simulink model "BMW"  (R2019b)
settings: Solver=VariableStepAuto  StartTime=0.0  StopTime=20  EnableMultiTasking=on
InitFcn:
  | % Modelisation de la Machine Synchrone
  | 
  | % Constantes
  | 
  | Rs = 0.001;
  | Rdd = 0.01 ;
  | Rdq = Rdd ;
  | Rf = 7 ;
  | Ld = 1.59e-2 ;
  | Lq = Ld ;
  | Lf = 7 ;
  | Ldd = 7e-4 ;
  | Ldq = Ldd ;
  | Maf = 0.259 ;
  | Madd = 2.5e-3 ;
  | Madq = Madd ;
  | Mfdd = 6.8e-2 ;
  | npp = 2 ;
  | J = 0.1 ;
  | 
  | m = 1.8e3;
  | g = 9.81;
  | Cr = 0.3;
  | rho = 1.225;
  | S = 2.25;
  | tau = 9.65;
  | Cx = 0.3;
  | Rw = 24.13e-2;
  | 
  | Jeq = 1;
  | feq = 1;
  | 
  | K = 0.5;
  | phi = 0.5;
  | 
  | w = 2*pi*50 ;
  | 
  | Omega = w/npp ;
  | 
  | 
  | % Matrices
  | 
  | % V = [Vd Vq 0 0 Vf] ;
  | 
  | % I = [Id Iq Idd Idq If] ;
  | 
  | % F = [Fd Fq Fdd Fdq Ff] ;
  | 
  | L = [ Ld			0		Madd		0			Maf ;
  |       0			Lq		0			Madq		0 			;
  |       1.5*Madd	0		Ldd		0			Mfdd ;
  |       0        1.5*Madq			0			Ldq	0 ;
  |       1.5*Maf	0		Mfdd		0			Lf ] ;
  | 
  | L1 = inv(L) ;
  | 
  | R = [ Rs 0  0   0   0 ;
  |       0  Rs 0   0   0 ;
  |       0  0  Rdd 0   0 ;
  |       0  0  0   Rdq 0 ;
  |       0  0  0   0   Rf ] ;
  | 
  | D = [ 0 -1 0 0 0 ;
  |        1  0 0 0 0 ;
  |        0  0 0 0 0 ;
  |        0  0 0 0 0 ;
  |        0  0 0 0 0 ] ;
  | 
  |     Cl = (1/3)*[ 2  -1      -1 ;
  |      	  	        0  sqrt(3) -sqrt(3) ;
  |                   1  1       1 ] ;
  | 
  |      Cl1 = inv(Cl);
  | 
  | 
  | 
  | Clark=2/3*[	1		-1/2		-1/2
  | 	        0		sqrt(3)/2	-sqrt(3)/2
  | 	        1/2		1/2		1/2		]
  | 
  | InvClark=inv(Clark)
  | 
  | LVIDE=[Ldd   Mfdd
  |         Mfdd    Lf];
  | L2=inv(LVIDE);
  | RVIDE=[Rdd   0
  |         0    Rf];
undefined symbols (not defined in the file or in its folder): sigbuilder_block
libraries: fl_lib x12, nesl_utility x9, sdl_lib x6, simulink x4
settings Model: Creator=arzande  LastModifiedBy=jpcanesin
settings SolverCC: ZeroCrossAlgorithm=Adaptive
settings DataIOCC: LimitDataPoints=on  SaveFormat=Array  SignalLoggingSaveFormat=ModelDataLogs  ReturnWorkspaceOutputs=off
settings OptimizationCC: ExpressionDepthLimit=2147483647  InitFltsAndDblsToZero=on  LifeSpan=inf
settings DebuggingCC: UnderspecifiedInitializationDetection=Classic  MergeDetectMultiDrivingBlocksExec=none  IgnoredZcDiagnostic=none  SolverPrmCheckMsg=warning  FcnCallInpInsideContextMsg=warning  AllowSymbolicDim=off  StateNameClashWarn=warning  SFUnexpectedBacktrackingDiag=warning  SFNoUnconditionalDefaultTransitionDiag=warning  SFExecutionAtInitializationDiag=none  ArithmeticOperatorsInVariantConditions=warning
settings HardwareCC: ProdBitPerPointer=32  ProdBitPerSizeT=32  ProdBitPerPtrDiffT=32  ProdLargestAtomicFloat=None  ProdIntDivRoundTo=Undefined  ProdEndianess=Unspecified  ProdWordSize=32  ProdHWDeviceType=32-bit Generic
settings ModelReferenceCC: PropagateSignalLabelsOutOfModel=off
settings SFSimCC: SimUseLocalCustomCode=off  CustomCodeUndefinedFunction=UseInterfaceOnly
settings RTWCC: RTWUseLocalCustomCode=off
settings CodeAppCC: StateflowObjectComments=on
settings GRTTargetCC: TargetLangStandard=C89/C90 (ANSI)  GeneratePreprocessorConditionals=Disable all  CombineOutputUpdateFcns=off  GRTInterface=on
settings ConfigComp: CovMetricSettings=dw  CovHtmlReporting=on  CovSaveCumulativeToWorkspaceVar=on  CovSaveSingleToWorkspaceVar=on  CovExternalEMLEnable=off

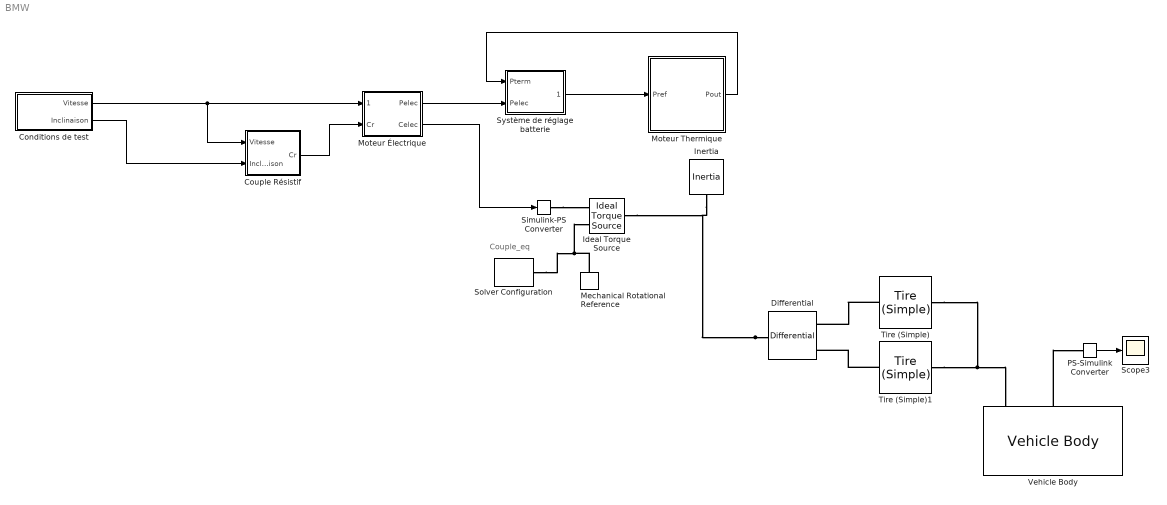
== system BMW ==
  note: Couple_eq
  Conditions de test : Subsystem  Tag=STV Subsys  LoadFcn=sigbuilder_block('load');  StartFcn=sigbuilder_block('start');  StopFcn=sigbuilder_block('stop');  ClipboardFcn=sigbuilder_block('clipboard');  mask(Sigbuilder block){tuvar=[0:10]}
      mask help: Simulink:masks:SigbuilderBlock_MD
      mask init:
      | if ~strcmp(get_param(bdroot(gcbh),'SimulationStatus'),'stopped') tuvar = sigbuilder_block('maskInit'); end
      settings: CopyFcn=sigbuilder_block('copy');  DeleteFcn=sigbuilder_block('delete');  ModelCloseFcn=sigbuilder_block('modelClose');  PreSaveFcn=sigbuilder_block('preSave');  PauseFcn=sigbuilder_block('pause');  ContinueFcn=sigbuilder_block('continue');  NameChangeFcn=sigbuilder_block('namechange');  OpenFcn=sigbuilder_block('open',[0 0 1396 804 ]);  CloseFcn=sigbuilder_block('close');
      mask Display: plot(0, 0, 100, 100,[2, 2, 32, 32, 2], [68, 8, 8, 68, 68],[32, 2], [38, 38], [32, 19, 2],[53, 60, 44], [32, 17, 17, 2],[16, 16, 31, 31]);txt = getActiveGroup(gcbh);text(2, 100, txt,'verticalAlignment', 'top');
  Couple Résistif : Subsystem
  Differential : sdl_lib/Gears/Differential  driveshaft_location=2  cd_ratio=4  friction_model=1  efficiency=[.85, .92]  mu_visc=[0, 0] N*m/(rad/s)  pwr_thr=[.001, .001] W  carrier_inertia=0 kg*m^2  planet_inertia=0 kg*m^2  temperature_TLU=[280, 300, 320] K  efficiency_ss_TLU=[.95, .9, .85]  efficiency_cd_TLU=[.95, .9, .85]  thermal_mass=50 J/K  T_init=300 K
      settings: SourceProductName=Simscape Driveline  SourceProductBaseCode=LD
  Ideal Torque Source : fl_lib/Mechanical/Mechanical Sources/Ideal Torque Source
  Inertia : fl_lib/Mechanical/Rotational Elements/Inertia  inertia=0.01 kg*m^2  w_specify=off  w_priority=High  w=0 rad/s  w_nominal_specify=off  w_nominal_unit=rad/s  w_nominal_value=1  t_specify=off  t_priority=None  t=0 N*m  t_nominal_specify=off  t_nominal_unit=N*m  t_nominal_value=1
  Mechanical Rotational Reference : fl_lib/Mechanical/Rotational Elements/Mechanical Rotational Reference
  Moteur Thermique : Subsystem
  Moteur Électrique : Subsystem
  PS-Simulink Converter : nesl_utility/PS-Simulink Converter  PhysicalDomain=network_engine_domain  SubClassName=ps_output  LeftPortType=input  RightPortType=output  PseudoPeriodic=off  Frequencies=[]  Unit=inherit  AffineConversion=off
  Scope3 : Scope
  Simulink-PS Converter : nesl_utility/Simulink-PS Converter  PhysicalDomain=network_engine_domain  SubClassName=ps_input  LeftPortType=input  RightPortType=output  PseudoPeriodic=off  Frequencies=[]  NoiseDistribution=none  NoiseParameters=[]  Unit=1  AffineConversion=off  FilteringAndDerivatives=provide  SimscapeFilterOrder=1  InputFilterTimeConstant=0.001  UdotUserProvided=0
  Solver Configuration : nesl_utility/Solver Configuration  PhysicalDomain=network_engine_domain  SubClassName=solver  LeftPortType=input  RightPortType=generic  Tones=[]  Harmonics=[]  SimulateNoise=off  Profile=off  UseLocalSampling=off  EnableSwitchedLinearOptims=on  FrequencyDomain=off  UseCCode=off  RelTol=0.001  AbsTol=1e-06  MinStep=1e-09  ToWorkspace=off  RevertToSquareIcSolve=off  NumHomotopyIterations=100  PhasorMode=off  PhasorModeNumHarmonics=1  DoDC=off  ResidualTolerance=1e-09  UseLocalSolver=off  LocalSolverChoice=NE_BACKWARD_EULER_ADVANCER  LocalSolverSampleTime=0.001  DoFixedCost=off  MaxNonlinIter=3  MaxModeIter=2  LinearAlgebra=auto  EquationFormulation=NE_TIME_EF  DelaysMemoryBudget=1024  AutomaticFiltering=on  FilteringTimeConstant=0.001  PartitionStorageMethod=AS_NEEDED  PartitionMemoryBudget=1024  PartitionMethod=ROBUST
  Système de réglage batterie : Subsystem
  Tire (Simple) : sdl_lib/Tires & Vehicles/Tire (Simple)  r_tire=0.3 m  model_compliance=0  stiffness=1e6 N/m  damping=1000 N/(m/s)  model_inertia=0  tire_inertia=1 kg*m^2  initial_velocity=0 rad/s
      settings: SourceProductName=Simscape Driveline  SourceProductBaseCode=LD  InternalSimscapePortConfiguration="{\"Bottom\":[],\"Left\":[{\"id\":\"A\",\"label\":\"A\",\"type\":\"foundation.mechanical.rotational.rotational\"}],\"Right\":[{\"id\":\"H\",\"label\":\"H\",\"type\":\"foundation.mechanical.translational.translational\"}],\"Top\":[]}"
  Tire (Simple)1 : sdl_lib/Tires & Vehicles/Tire (Simple)  r_tire=0.3 m  model_compliance=0  stiffness=1e6 N/m  damping=1000 N/(m/s)  model_inertia=0  tire_inertia=1 kg*m^2  initial_velocity=0 rad/s
      settings: SourceProductName=Simscape Driveline  SourceProductBaseCode=LD  InternalSimscapePortConfiguration="{\"Bottom\":[],\"Left\":[{\"id\":\"A\",\"label\":\"A\",\"type\":\"foundation.mechanical.rotational.rotational\"}],\"Right\":[{\"id\":\"H\",\"label\":\"H\",\"type\":\"foundation.mechanical.translational.translational\"}],\"Top\":[]}"
  Vehicle Body : sdl_lib/Tires & Vehicles/Vehicle Body  mass=1200 kg  n_w=2  x_f=1.4 m  x_r=1.6 m  y_c=0.5 m  mass_var=simscape.enum.onoff.off  model_pitch=simscape.enum.onoff.off  inertia=4000 kg*m^2  suspension_model=sdl.enum.linearTLU.linear  k_f=1e4 N/m  b_f=1e4 N/(m/s)  k_r=1e4 N/m  b_r=1e4 N/(m/s)  k_f_TLU=[-2000, -1000, 0, 1000, 2000] N  x_f_TLU=[-.4, -.2, 0, .2, .4] m  b_f_TLU=[-200, -100, 0, 100, 200] N  v_f_TLU=[-4, -2, 0, 2, 4] m/s  k_r_TLU=[-2000, -1000, 0, 1000, 2000] N  x_r_TLU=[-.4, -.2, 0, .2, .4] m  b_r_TLU=[-200, -100, 0, 100, 200] N  v_r_TLU=[-4, -2, 0, 2, 4] m/s  interp_method=simscape.enum.interpolation.linear  extrap_method=simscape.enum.extrapolation.linear  model_hardstop=simscape.enum.onoff.off  upper_bound_f=.25 m  lower_bound_f=-.25 m  stop_k_f=1e6 N/m  stop_b_f=150 N/(m/s)  upper_bound_r=.25 m  lower_bound_r=-.25 m  stop_k_r=1e6 N/m  stop_b_r=150 N/(m/s)  initial_pitch=0 rad  initial_pitch_rate=0 rad/s  g=9.81 m/s^2  liftoff_warning=simscape.enum.onoff.off  area=3 m^2  Cd=0.4  rho=1.18 kg/m^3  v_specify=on  v_priority=None  v=0 m/s  v_nominal_specify=off  v_nominal_unit=m/s  v_nominal_value=1
      settings: SourceProductName=Simscape Driveline
  wires:
  Conditions de test/1(Vitesse) -> Couple Résistif/1(Vitesse), Moteur Électrique/1(Vitesse)
  PS-Simulink Converter/1 -> Scope3/1
  Conditions de test/2(Inclinaison) -> Couple Résistif/2(Inclinaison)
  Couple Résistif/1(Cr) -> Moteur Électrique/2(Cr)
  Moteur Électrique/2(Celec) -> Simulink-PS Converter/1
  Moteur Thermique/1(Pout) -> Système de réglage batterie/1(Pterm)
  Moteur Électrique/1(Pelec) -> Système de réglage batterie/2(Pelec)
  Système de réglage batterie/1(Pterm_ref) -> Moteur Thermique/1(Pref)
  connections:
  Tire (Simple)1/RConn1 -- Tire (Simple)/RConn1 -- Vehicle Body/LConn1
  Differential/LConn1 -- Inertia/LConn1 -- Ideal Torque Source/LConn1
  Tire (Simple)1/LConn1 -- Differential/RConn1
  Vehicle Body/LConn2 -- PS-Simulink Converter/LConn1
  Tire (Simple)/LConn1 -- Differential/RConn2
  Simulink-PS Converter/RConn1 -- Ideal Torque Source/RConn1
  Mechanical Rotational Reference/LConn1 -- Solver Configuration/RConn1 -- Ideal Torque Source/RConn2

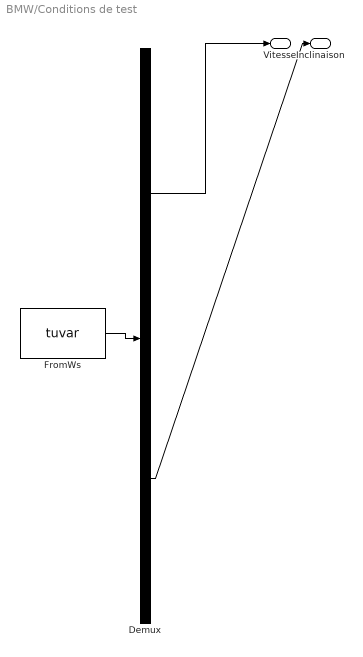
== system BMW/Conditions de test ==
  Demux : Demux  Tag=STV Demux  Outputs=2
  FromWs : FromWorkspace  Tag=STV FromWs  VariableName=tuvar  SampleTime=0
      SigBuilderData=|
      | common.afterFinalStr = 'Extrapolate'
      | common.sampleTime = 0
      | dataSet.timeRange = [0 10]
      | dataSet.name = 'Group 1'
      | sbobj.Groups.Name = 'Group 1'
      | sbobj.Groups.Signals(1).Name = 'Vitesse'
      | sbobj.Groups.Signals(1).XData = [0 4 10]
      | sbobj.Groups.Signals(1).YData = [0 25 25]
      | sbobj.Groups.Signals(2).Name = 'Inclinaison'
      | sbobj.Groups.Signals(2).XData = [0 2.96 6.75 9.86 10]
      | sbobj.Groups.Signals(2).YData = [0 0 0 0 0]
  Vitesse : Outport  Tag=STV Outport
  Inclinaison : Outport  Tag=STV Outport  Port=2
  wires:
  Demux/1 -> Vitesse/1
  FromWs/1 -> Demux/1
  Demux/2 -> Inclinaison/1

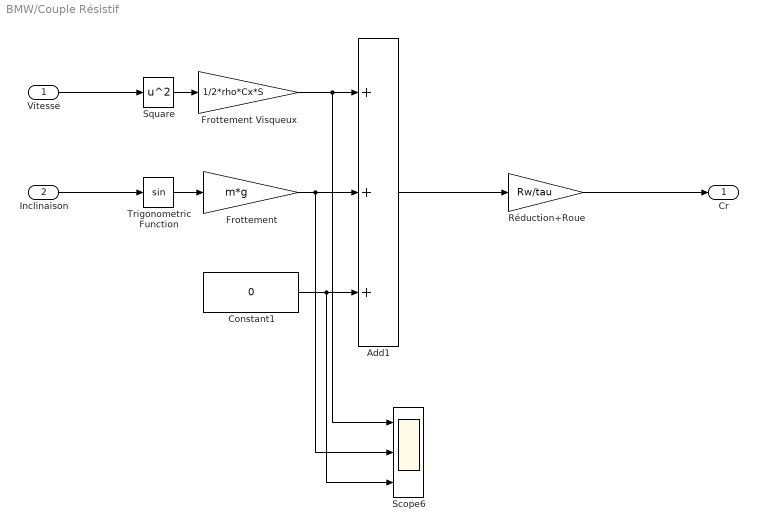
== system BMW/Couple Résistif ==
  Vitesse : Inport
  Inclinaison : Inport  Port=2
  Add1 : Sum  Inputs=+++
  Constant1 : Constant  Value=0
  "Frottement " : Gain  Gain=m*g
  Frottement Visqueux : Gain  Gain=1/2*rho*Cx*S
  Réduction+Roue : Gain  Gain=Rw/tau
  Scope6 : Scope  NumInputPorts=3
  Square : Math  Operator=square  SignedPower=off  SaturateOnIntegerOverflow=on
  Trigonometric Function : Trigonometry
  Cr : Outport
  wires:
  Réduction+Roue/1 -> Cr/1
  Add1/1 -> Réduction+Roue/1
  Trigonometric Function/1 -> "Frottement "/1
  Inclinaison/1 -> Trigonometric Function/1
  Vitesse/1 -> Square/1
  Constant1/1 -> Scope6/3, Add1/3
  Square/1 -> Frottement Visqueux/1
  Frottement Visqueux/1 -> Scope6/1, Add1/1
  "Frottement "/1 -> Scope6/2, Add1/2

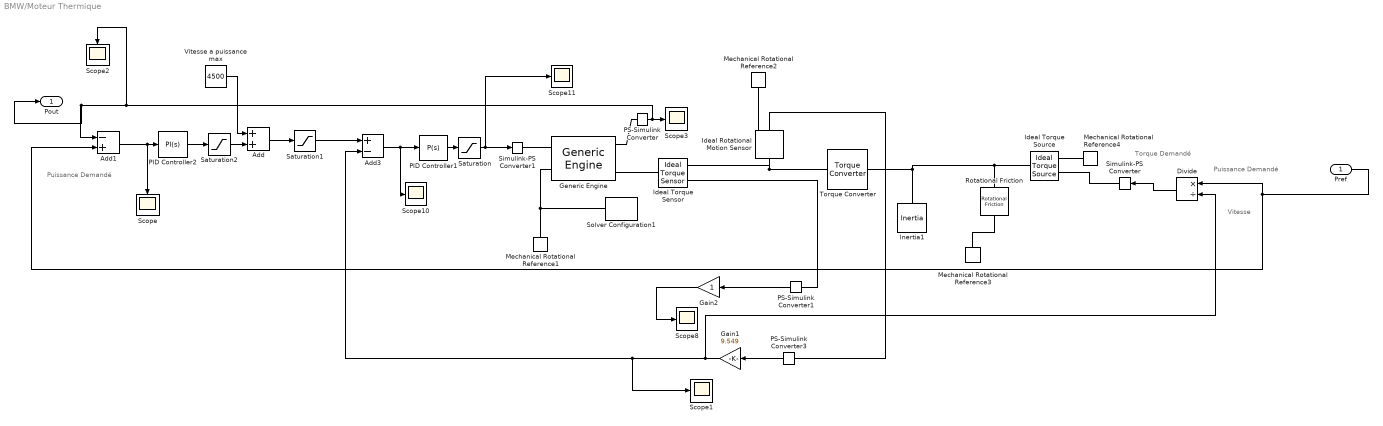
== system BMW/Moteur Thermique ==
  note: Vitesse
  note: Torque Demandé
  note: Puissance Demandé
  note: Puissance Demandé
  Pref : Inport
  Add : Sum
  Add1 : Sum  Inputs=-+
  Add3 : Sum  Inputs=+-
  Divide : Product  Inputs=*/
  Gain1 : Gain  Gain=9.549
  Gain2 : Gain
  Generic Engine : sdl_lib/Engines/Generic Engine  model_parameterization=1  engine_type=1  P_max=150 kW  w_P_max=4500 rpm  w_max=7000 rpm  w_min=800 rpm  w_tab=[500, 1000, 2000, 3000, 4000, 5000, 6000, 7000] rpm  trq_tab=[380, 380, 380, 380, 350, 280, 200, 80] N*m  pwr_tab=[20, 40, 78, 120, 145, 148, 125, 60] kW  interp_method=simscape.enum.interpolation.linear  model_inertia=1  inertia=0.2 kg*m^2  initial_velocity=800 rpm  model_time_constant=0  time_constant=0.2 s  T0=0  w_thr=100 rpm  idle_speed=0  idle_speed_reference=1000 rpm  tau_controller=1 s  idle_w_thr=1 rpm  redline=0  redline_speed=5000 rpm  tau_redline=1 s  redline_w_thr=1 rpm  fc_model=0  fc_per_rev=25 mg/rev  displaced_volume=400 cm^3  rev_per_cycle=2  fc_w_tab=[1000, 2000, 3000, 4000, 5000, 6000] rpm  fc_trq_tab=[0, 80, 160, 200, 240, 320, 360, 400] N*m  fc_tab=[.5, .9, 1.4, 1.6, 1.9, 2.7, 3.4, 4.4; 1, 1.7, 2.7, 3.1, 3.6, 5, 6, 7.4; 1.4, 2.7, 4, 4.8, 5.6, 7.5, 8.5, 10.5; 2, 3.6, 5.8, 6.7, 8, 10.4, 11.7, 13.3; 2.5, 4.8, 7.9, 9.4, 10.8, 14, 16.2, 18.6; 3.1, 6, 10.3, 11.9, 13.8, 18.4, 22, 26.5] g/s  bmep_tab=[0, 250, 500, 625, 750, 1000, 1150, 1250] kPa  bsfc_tab=[410, 380, 300, 280, 270, 290, 320, 380; 410, 370, 290, 270, 260, 270, 285, 320; 415, 380, 290, 275, 265, 270, 270, 300; 420, 390, 310, 290, 285, 280, 280, 285; 430, 410, 340, 320, 310, 300, 310, 320; 450, 430, 370, 340, 330, 330, 350, 380] g/hr/kW  fc_interp_method=simscape.enum.interpolation.linear
      settings: SourceProductName=Simscape Driveline  SourceProductBaseCode=LD  InternalSimscapePortConfiguration="{\"Bottom\":[],\"Left\":[{\"id\":\"T\",\"label\":\"T\",\"type\":\"input\"},{\"id\":\"B\",\"label\":\"B\",\"type\":\"foundation.mechanical.rotational.rotational\"}],\"Right\":[{\"id\":\"P\",\"label\":\"P\",\"type\":\"output\"},{\"id\":\"FC\",\"label\":\"FC\",\"type\":\"output\"},{\"id\":\"F\",\"label\":\"F\",\"type\":\"foundation.mechanical.rotational.rotational\"}],\"Top\":[]}"
  Ideal Rotational Motion Sensor : fl_lib/Mechanical/Mechanical Sensors/Ideal Rotational Motion Sensor  offset=0 rad
  Ideal Torque Sensor : fl_lib/Mechanical/Mechanical Sensors/Ideal Torque Sensor
  Ideal Torque Source : fl_lib/Mechanical/Mechanical Sources/Ideal Torque Source
  Inertia1 : fl_lib/Mechanical/Rotational Elements/Inertia  inertia=1 kg*m^2  w_specify=off  w_priority=High  w=0 rad/s  w_nominal_specify=off  w_nominal_unit=rad/s  w_nominal_value=1  t_specify=off  t_priority=None  t=0 N*m  t_nominal_specify=off  t_nominal_unit=N*m  t_nominal_value=1
  Mechanical Rotational Reference{1..4} (4 alike) : fl_lib/Mechanical/Rotational Elements/Mechanical Rotational Reference
  PID Controller1 : simulink/Continuous/PID Controller  Controller=P  Form=Parallel  TimeDomain=Continuous-time  SampleTime=-1  IntegratorMethod=Forward Euler  FilterMethod=Forward Euler  ControllerParametersSource=internal  P=.1  I=1  D=0  UseFilter=on  N=100  TunerSelectOption=Transfer Function Based (PID Tuner App)  InitialConditionSource=internal  InitialConditionForIntegrator=0  InitialConditionForFilter=0  DifferentiatorICPrevScaledInput=0  ExternalReset=none  TrackingMode=off  Kt=1  LimitOutput=off  UpperSaturationLimit=inf  LowerSaturationLimit=-inf  LinearizeAsGain=on  AntiWindupMode=none  Kb=1  POutMin=[]  POutMax=[]  IOutMin=[]  IOutMax=[]  DOutMin=[]  DOutMax=[]  NOutMin=[]  NOutMax=[]  SumOutMin=[]  SumOutMax=[]  SaturationOutMin=[]  SaturationOutMax=[]  PParamMin=[]  PParamMax=[]  IParamMin=[]  IParamMax=[]  DParamMin=[]  DParamMax=[]  NParamMin=[]  NParamMax=[]  KbParamMin=[]  KbParamMax=[]  KtParamMin=[]  KtParamMax=[]  KbOutMin=[]  KbOutMax=[]  KtOutMin=[]  KtOutMax=[]  IntegratorOutMin=[]  IntegratorOutMax=[]  FilterOutMin=[]  FilterOutMax=[]  SumI1OutMin=[]  SumI1OutMax=[]  SumI2OutMin=[]  SumI2OutMax=[]  SumI3OutMin=[]  SumI3OutMax=[]  SumI4OutMin=[]  SumI4OutMax=[]  SumDOutMin=[]  SumDOutMax=[]  DifferentiatorOutMin=[]  DifferentiatorOutMax=[]  FilterDiffOutCoefMin=[]  FilterDiffOutCoefMax=[]  ReciprocalOutMin=[]  ReciprocalOutMax=[]  SumDenOutMin=[]  SumDenOutMax=[]  SumNumOutMin=[]  SumNumOutMax=[]  DivideOutMin=[]  DivideOutMax=[]  IntegratorContinuousStateAttributes=''  IntegratorStateMustResolveToSignalObject=off  IntegratorRTWStateStorageClass=Auto  FilterContinuousStateAttributes=''  FilterStateMustResolveToSignalObject=off  FilterRTWStateStorageClass=Auto  ParallelPVariant=InternalParameters  IdealPVariant=Disabled  IVariant=Disabled  DVariant=Disabled  IntegratorVariant=Disabled  SatVariant=Disabled  AWVariant=Disabled  PCopyVariant=Disabled  TRVariant=Disabled  FdbkBlocksVariant=Forward  IdealPFdbkVariant=Disabled  SatFdbkVariant=Disabled  DerivativeFilterVariant=Disabled  NVariant=Disabled  NCopyVariant=Disabled_SignalSpec  FilterICVariant=Disabled  IntegratorICVariant=Disabled  ExternalResetVariant=Disabled  TRSumVariant=Passthrough  SumFdbkVariant=Disabled  SumVariant=Passthrough_P
  PID Controller2 : simulink/Continuous/PID Controller  Controller=PI  Form=Parallel  TimeDomain=Continuous-time  SampleTime=-1  IntegratorMethod=Forward Euler  FilterMethod=Forward Euler  ControllerParametersSource=internal  P=1  I=1  D=0  UseFilter=on  N=100  TunerSelectOption=Transfer Function Based (PID Tuner App)  InitialConditionSource=internal  InitialConditionForIntegrator=0  InitialConditionForFilter=0  DifferentiatorICPrevScaledInput=0  ExternalReset=none  TrackingMode=off  Kt=1  LimitOutput=off  UpperSaturationLimit=inf  LowerSaturationLimit=-inf  LinearizeAsGain=on  AntiWindupMode=none  Kb=1  POutMin=[]  POutMax=[]  IOutMin=[]  IOutMax=[]  DOutMin=[]  DOutMax=[]  NOutMin=[]  NOutMax=[]  SumOutMin=[]  SumOutMax=[]  SaturationOutMin=[]  SaturationOutMax=[]  PParamMin=[]  PParamMax=[]  IParamMin=[]  IParamMax=[]  DParamMin=[]  DParamMax=[]  NParamMin=[]  NParamMax=[]  KbParamMin=[]  KbParamMax=[]  KtParamMin=[]  KtParamMax=[]  KbOutMin=[]  KbOutMax=[]  KtOutMin=[]  KtOutMax=[]  IntegratorOutMin=[]  IntegratorOutMax=[]  FilterOutMin=[]  FilterOutMax=[]  SumI1OutMin=[]  SumI1OutMax=[]  SumI2OutMin=[]  SumI2OutMax=[]  SumI3OutMin=[]  SumI3OutMax=[]  SumI4OutMin=[]  SumI4OutMax=[]  SumDOutMin=[]  SumDOutMax=[]  DifferentiatorOutMin=[]  DifferentiatorOutMax=[]  FilterDiffOutCoefMin=[]  FilterDiffOutCoefMax=[]  ReciprocalOutMin=[]  ReciprocalOutMax=[]  SumDenOutMin=[]  SumDenOutMax=[]  SumNumOutMin=[]  SumNumOutMax=[]  DivideOutMin=[]  DivideOutMax=[]  IntegratorContinuousStateAttributes=''  IntegratorStateMustResolveToSignalObject=off  IntegratorRTWStateStorageClass=Auto  FilterContinuousStateAttributes=''  FilterStateMustResolveToSignalObject=off  FilterRTWStateStorageClass=Auto  ParallelPVariant=InternalParameters  IdealPVariant=Disabled  IVariant=InternalParameters  DVariant=Disabled  IntegratorVariant=Continuous  SatVariant=Disabled  AWVariant=Passthrough  PCopyVariant=Disabled  TRVariant=Disabled  FdbkBlocksVariant=Forward  IdealPFdbkVariant=Disabled  SatFdbkVariant=Disabled  DerivativeFilterVariant=Disabled  NVariant=Disabled  NCopyVariant=Disabled_SignalSpec  FilterICVariant=Disabled  IntegratorICVariant=InternalICs  ExternalResetVariant=Disabled  TRSumVariant=Passthrough  SumFdbkVariant=Disabled  SumVariant=Sum_PI
  PS-Simulink Converter : nesl_utility/PS-Simulink Converter  PhysicalDomain=network_engine_domain  SubClassName=ps_output  LeftPortType=input  RightPortType=output  PseudoPeriodic=off  Frequencies=[]  Unit=inherit  AffineConversion=off
  PS-Simulink Converter1 : nesl_utility/PS-Simulink Converter  PhysicalDomain=network_engine_domain  SubClassName=ps_output  LeftPortType=input  RightPortType=output  PseudoPeriodic=off  Frequencies=[]  Unit=inherit  AffineConversion=off
  PS-Simulink Converter3 : nesl_utility/PS-Simulink Converter  PhysicalDomain=network_engine_domain  SubClassName=ps_output  LeftPortType=input  RightPortType=output  PseudoPeriodic=off  Frequencies=[]  Unit=inherit  AffineConversion=off
  Rotational Friction : fl_lib/Mechanical/Rotational Elements/Rotational Friction  brkwy_trq=25 N*m  brkwy_vel=0.1 rad/s  Col_trq=20 N*m  visc_coef=0.001 N*m/(rad/s)  w_specify=off  w_priority=None  w=0 rad/s  w_nominal_specify=off  w_nominal_unit=rad/s  w_nominal_value=1  t_specify=off  t_priority=None  t=0 N*m  t_nominal_specify=off  t_nominal_unit=N*m  t_nominal_value=1
      settings: SourceProductName=Simscape
  Saturation : Saturate  UpperLimit=1  LowerLimit=0
  Saturation1 : Saturate  UpperLimit=6999  LowerLimit=0
  Saturation2 : Saturate  UpperLimit=0  LowerLimit=-4500
  Scope{,1..3,8,10..11} (7 alike) : Scope
  Simulink-PS Converter : nesl_utility/Simulink-PS Converter  PhysicalDomain=network_engine_domain  SubClassName=ps_input  LeftPortType=input  RightPortType=output  PseudoPeriodic=off  Frequencies=[]  NoiseDistribution=none  NoiseParameters=[]  Unit=1  AffineConversion=off  FilteringAndDerivatives=provide  SimscapeFilterOrder=1  InputFilterTimeConstant=0.001  UdotUserProvided=0
  Simulink-PS Converter1 : nesl_utility/Simulink-PS Converter  PhysicalDomain=network_engine_domain  SubClassName=ps_input  LeftPortType=input  RightPortType=output  PseudoPeriodic=off  Frequencies=[]  NoiseDistribution=none  NoiseParameters=[]  Unit=1  AffineConversion=off  FilteringAndDerivatives=provide  SimscapeFilterOrder=1  InputFilterTimeConstant=0.001  UdotUserProvided=0
  Solver Configuration1 : nesl_utility/Solver Configuration  PhysicalDomain=network_engine_domain  SubClassName=solver  LeftPortType=input  RightPortType=generic  Tones=[]  Harmonics=[]  SimulateNoise=off  Profile=off  UseLocalSampling=off  EnableSwitchedLinearOptims=on  FrequencyDomain=off  UseCCode=off  RelTol=0.001  AbsTol=1e-06  MinStep=1e-09  ToWorkspace=off  RevertToSquareIcSolve=off  NumHomotopyIterations=100  PhasorMode=off  PhasorModeNumHarmonics=1  DoDC=off  ResidualTolerance=1e-09  UseLocalSolver=off  LocalSolverChoice=NE_BACKWARD_EULER_ADVANCER  LocalSolverSampleTime=0.001  DoFixedCost=off  MaxNonlinIter=3  MaxModeIter=2  LinearAlgebra=auto  EquationFormulation=NE_TIME_EF  DelaysMemoryBudget=1024  AutomaticFiltering=on  FilteringTimeConstant=0.001  PartitionStorageMethod=AS_NEEDED  PartitionMemoryBudget=1024  PartitionMethod=ROBUST
  Torque Converter : sdl_lib/Couplings & Drives/Torque Converter  n_vector=[0, .5, .6, .7, .8, .87, .92, .94, .96, .97]  trq_vector=[2.232, 1.5462, 1.4058, 1.2746, 1.1528, 1.0732, 1.0192, .9983, .9983, .9983]  cf_vector_parameterization=1  cf_vector_reference_speed=1  cf_vector=[12.2938, 12.8588, 13.1452, 13.6285, 14.6163, 16.2675, 19.3503, 22.1046, 29.9986, 50] (rad/s)/(N*m)^0.5  cf_vector_sq=1e-3 * [6.616, 6.048, 5.787, 5.384, 4.681, 3.779, 2.671, 2.047, 1.111, .4] N*m/(rad/s)^2  interp_method=simscape.enum.interpolation.linear  extrap_method=simscape.enum.extrapolation.linear  model_lag=1  tau=.02 s  initial_trq_ratio=0
      settings: SourceProductName=Simscape Driveline  SourceProductBaseCode=LD  InternalSimscapePortConfiguration="{\"Bottom\":[],\"Left\":[{\"id\":\"I\",\"label\":\"I\",\"type\":\"foundation.mechanical.rotational.rotational\"}],\"Right\":[{\"id\":\"T\",\"label\":\"T\",\"type\":\"foundation.mechanical.rotational.rotational\"}],\"Top\":[]}"
  Vitesse a puissance max : Constant  Value=4500
  Pout : Outport
  wires:
  PID Controller2/1 -> Saturation2/1
  Vitesse a puissance max/1 -> Add/1
  PS-Simulink Converter1/1 -> Gain2/1
  Saturation1/1 -> Add3/1
  Saturation/1 -> Simulink-PS Converter1/1, Scope11/1
  Gain2/1 -> Scope8/1
  Add1/1 -> Scope/1, PID Controller2/1
  PID Controller1/1 -> Saturation/1
  Saturation2/1 -> Add/2
  Gain1/1 -> Divide/2, Add3/2, Scope1/1
  PS-Simulink Converter3/1 -> Gain1/1
  Divide/1 -> Simulink-PS Converter/1
  Pref/1 -> Divide/1, Add1/2
  Add/1 -> Saturation1/1
  Add3/1 -> Scope10/1, PID Controller1/1
  PS-Simulink Converter/1 -> Scope2/1, Pout/1, Add1/1, Scope3/1
  connections:
  PS-Simulink Converter1/LConn1 -- Ideal Torque Sensor/RConn2
  Mechanical Rotational Reference4/LConn1 -- Ideal Torque Source/RConn2
  Generic Engine/LConn1 -- Simulink-PS Converter1/RConn1
  Ideal Rotational Motion Sensor/LConn1 -- Torque Converter/LConn1 -- Ideal Torque Sensor/RConn1
  Mechanical Rotational Reference2/LConn1 -- Ideal Rotational Motion Sensor/RConn1
  Ideal Torque Source/RConn1 -- Simulink-PS Converter/RConn1
  Generic Engine/LConn2 -- Solver Configuration1/RConn1 -- Mechanical Rotational Reference1/LConn1
  Ideal Rotational Motion Sensor/RConn2 -- PS-Simulink Converter3/LConn1
  Mechanical Rotational Reference3/LConn1 -- Rotational Friction/RConn1
  Torque Converter/RConn1 -- Inertia1/LConn1 -- Ideal Torque Source/LConn1 -- Rotational Friction/LConn1
  Ideal Torque Sensor/LConn1 -- Generic Engine/RConn3
  Generic Engine/RConn1 -- PS-Simulink Converter/LConn1

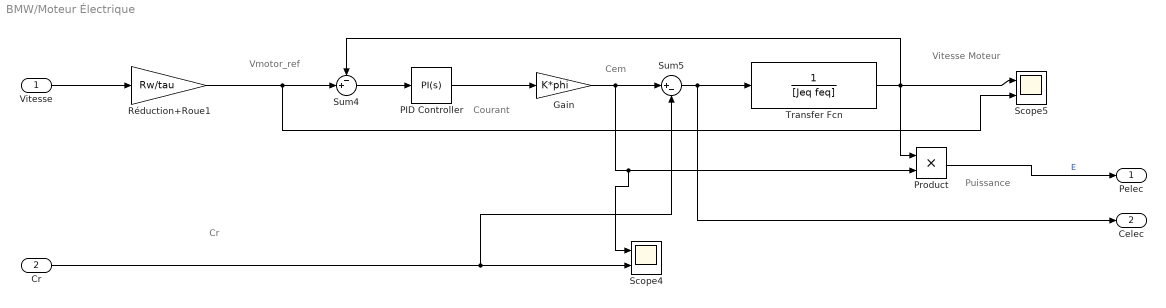
== system BMW/Moteur Électrique ==
  note: Puissance
  note: Vitesse Moteur
  note: Courant
  note: Vmotor_ref
  note: Cem
  note: Cr
  Vitesse : Inport
  Cr : Inport  Port=2
  Gain : Gain  Gain=K*phi
  PID Controller : simulink/Continuous/PID Controller  Controller=PI  Form=Parallel  TimeDomain=Continuous-time  SampleTime=-1  IntegratorMethod=Forward Euler  FilterMethod=Forward Euler  ControllerParametersSource=internal  P=2000  I=2000*feq/Jeq  D=0  UseFilter=on  N=100  TunerSelectOption=Transfer Function Based (PID Tuner App)  InitialConditionSource=internal  InitialConditionForIntegrator=0  InitialConditionForFilter=0  DifferentiatorICPrevScaledInput=0  ExternalReset=none  TrackingMode=off  Kt=1  LimitOutput=off  UpperSaturationLimit=inf  LowerSaturationLimit=-inf  LinearizeAsGain=on  AntiWindupMode=none  Kb=1  POutMin=[]  POutMax=[]  IOutMin=[]  IOutMax=[]  DOutMin=[]  DOutMax=[]  NOutMin=[]  NOutMax=[]  SumOutMin=[]  SumOutMax=[]  SaturationOutMin=[]  SaturationOutMax=[]  PParamMin=[]  PParamMax=[]  IParamMin=[]  IParamMax=[]  DParamMin=[]  DParamMax=[]  NParamMin=[]  NParamMax=[]  KbParamMin=[]  KbParamMax=[]  KtParamMin=[]  KtParamMax=[]  KbOutMin=[]  KbOutMax=[]  KtOutMin=[]  KtOutMax=[]  IntegratorOutMin=[]  IntegratorOutMax=[]  FilterOutMin=[]  FilterOutMax=[]  SumI1OutMin=[]  SumI1OutMax=[]  SumI2OutMin=[]  SumI2OutMax=[]  SumI3OutMin=[]  SumI3OutMax=[]  SumI4OutMin=[]  SumI4OutMax=[]  SumDOutMin=[]  SumDOutMax=[]  DifferentiatorOutMin=[]  DifferentiatorOutMax=[]  FilterDiffOutCoefMin=[]  FilterDiffOutCoefMax=[]  ReciprocalOutMin=[]  ReciprocalOutMax=[]  SumDenOutMin=[]  SumDenOutMax=[]  SumNumOutMin=[]  SumNumOutMax=[]  DivideOutMin=[]  DivideOutMax=[]  IntegratorContinuousStateAttributes=''  IntegratorStateMustResolveToSignalObject=off  IntegratorRTWStateStorageClass=Auto  FilterContinuousStateAttributes=''  FilterStateMustResolveToSignalObject=off  FilterRTWStateStorageClass=Auto  ParallelPVariant=InternalParameters  IdealPVariant=Disabled  IVariant=InternalParameters  DVariant=Disabled  IntegratorVariant=Continuous  SatVariant=Disabled  AWVariant=Passthrough  PCopyVariant=Disabled  TRVariant=Disabled  FdbkBlocksVariant=Forward  IdealPFdbkVariant=Disabled  SatFdbkVariant=Disabled  DerivativeFilterVariant=Disabled  NVariant=Disabled  NCopyVariant=Disabled_SignalSpec  FilterICVariant=Disabled  IntegratorICVariant=InternalICs  ExternalResetVariant=Disabled  TRSumVariant=Passthrough  SumFdbkVariant=Disabled  SumVariant=Sum_PI
  Product : Product
  Réduction+Roue1 : Gain  Gain=Rw/tau
  Scope4 : Scope  NumInputPorts=2
  Scope5 : Scope  NumInputPorts=2
  Sum4 : Sum  Inputs=-+|  SaturateOnIntegerOverflow=on
  Sum5 : Sum  Inputs=|+-  SaturateOnIntegerOverflow=on
  Transfer Fcn : TransferFcn  Denominator=[Jeq feq]
  Pelec : Outport
  Celec : Outport  Port=2
  wires:
  Sum4/1 -> PID Controller/1
  Sum5/1 -> Celec/1, Transfer Fcn/1
  Transfer Fcn/1 -> Scope5/1, Product/1, Sum4/1
  Gain/1 -> Scope4/1, Product/2, Sum5/1
  Réduction+Roue1/1 -> Scope5/2, Sum4/2
  Product/1 -> Pelec/1  "E"
  Vitesse/1 -> Réduction+Roue1/1
  Cr/1 -> Sum5/2, Scope4/2
  PID Controller/1 -> Gain/1

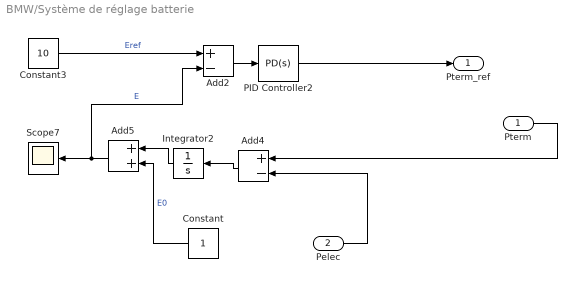
== system BMW/Système de réglage batterie ==
  Pterm : Inport
  Pelec : Inport  Port=2
  Add2 : Sum  Inputs=+-
  Add4 : Sum  Inputs=+-
  Add5 : Sum
  Constant : Constant
  Constant3 : Constant  Value=10
  Integrator2 : Integrator
  PID Controller2 : simulink/Continuous/PID Controller  Controller=PD  Form=Parallel  TimeDomain=Continuous-time  SampleTime=-1  IntegratorMethod=Forward Euler  FilterMethod=Forward Euler  ControllerParametersSource=internal  P=.1  I=1  D=0  UseFilter=on  N=100  TunerSelectOption=Transfer Function Based (PID Tuner App)  InitialConditionSource=internal  InitialConditionForIntegrator=0  InitialConditionForFilter=0  DifferentiatorICPrevScaledInput=0  ExternalReset=none  TrackingMode=off  Kt=1  LimitOutput=off  UpperSaturationLimit=inf  LowerSaturationLimit=-inf  LinearizeAsGain=on  AntiWindupMode=none  Kb=1  POutMin=[]  POutMax=[]  IOutMin=[]  IOutMax=[]  DOutMin=[]  DOutMax=[]  NOutMin=[]  NOutMax=[]  SumOutMin=[]  SumOutMax=[]  SaturationOutMin=[]  SaturationOutMax=[]  PParamMin=[]  PParamMax=[]  IParamMin=[]  IParamMax=[]  DParamMin=[]  DParamMax=[]  NParamMin=[]  NParamMax=[]  KbParamMin=[]  KbParamMax=[]  KtParamMin=[]  KtParamMax=[]  KbOutMin=[]  KbOutMax=[]  KtOutMin=[]  KtOutMax=[]  IntegratorOutMin=[]  IntegratorOutMax=[]  FilterOutMin=[]  FilterOutMax=[]  SumI1OutMin=[]  SumI1OutMax=[]  SumI2OutMin=[]  SumI2OutMax=[]  SumI3OutMin=[]  SumI3OutMax=[]  SumI4OutMin=[]  SumI4OutMax=[]  SumDOutMin=[]  SumDOutMax=[]  DifferentiatorOutMin=[]  DifferentiatorOutMax=[]  FilterDiffOutCoefMin=[]  FilterDiffOutCoefMax=[]  ReciprocalOutMin=[]  ReciprocalOutMax=[]  SumDenOutMin=[]  SumDenOutMax=[]  SumNumOutMin=[]  SumNumOutMax=[]  DivideOutMin=[]  DivideOutMax=[]  IntegratorContinuousStateAttributes=''  IntegratorStateMustResolveToSignalObject=off  IntegratorRTWStateStorageClass=Auto  FilterContinuousStateAttributes=''  FilterStateMustResolveToSignalObject=off  FilterRTWStateStorageClass=Auto  ParallelPVariant=InternalParameters  IdealPVariant=Disabled  IVariant=Disabled  DVariant=InternalParameters  IntegratorVariant=Disabled  SatVariant=Disabled  AWVariant=Disabled  PCopyVariant=Disabled  TRVariant=Disabled  FdbkBlocksVariant=Forward  IdealPFdbkVariant=Disabled  SatFdbkVariant=Disabled  DerivativeFilterVariant=ContFilter  NVariant=InternalParameters  NCopyVariant=Disabled  FilterICVariant=InternalICsFilter  IntegratorICVariant=Disabled  ExternalResetVariant=Disabled  TRSumVariant=Passthrough  SumFdbkVariant=Disabled  SumVariant=Sum_PD
  Scope7 : Scope
  Pterm_ref : Outport
  wires:
  Pterm/1 -> Add4/1
  PID Controller2/1 -> Pterm_ref/1
  Constant3/1 -> Add2/1  "Eref"
  Add2/1 -> PID Controller2/1
  Integrator2/1 -> Add5/1
  Constant/1 -> Add5/2  "E0"
  Add5/1 -> Add2/2, Scope7/1  "E"
  Pelec/1 -> Add4/2
  Add4/1 -> Integrator2/1
